simulink model "PenduloRotativoSim"  (R2025a)
settings: Solver=VariableStepAuto  StartTime=0.0  StopTime=4  FixedStep=0.002  RelTol=1e-3  EnableMultiTasking=on
undefined symbols (not defined in the file): K, Ts, x_ic, xp_ic
settings Model: SimulationMode=external  ExtModeTrigDuration=10000  Creator=aluno.engenharia  LastModifiedBy=Mateus
settings SolverCC: AlgebraicLoopSolver=TrustRegion  PositivePriorityOrder=on
settings DebuggingCC: UnconnectedInputMsg=warning  UnconnectedOutputMsg=warning  UnconnectedLineMsg=warning
settings ModelReferenceCC: EnableRefExpFcnMdlSchedulingChecks=on
settings SFSimCC: CustomCodeUndefinedFunction=UseInterfaceOnly
settings RTWCC: SystemTargetFile=quarc_win64.tlc  TemplateMakefile=quarc_default_tmf  GPUComputeCapability=3.5  Description=QUARC Win64 Target
settings STFCustomTargetCC: SystemTargetFile=quarc_win64.tlc  TargetPreCompLibLocation=C:\PROGRA~3\QUARC\lib\2019a\win64\release  TargetLangStandard=C99 (ISO)  MultiwordLength=2048.0  DynamicStringBufferSize=256.0  ConcurrentExecutionCompliant=on  StopOnOverrun=off  DownloadToTarget=on  Debug=off
settings GRTTargetCC: ExtMode=on  ExtModeMexFile=quarc_comm  TargetPreCompLibLocation=C:\PROGRA~3\QUARC\lib\2019a\win64\release  ParMdlRefBuildCompliant=off  CompOptLevelCompliant=off  CombineOutputUpdateFcns=off  MatFileLogging=off  CPPClassGenCompliant=off  GRTInterface=on  UseToolchainInfoCompliant=off

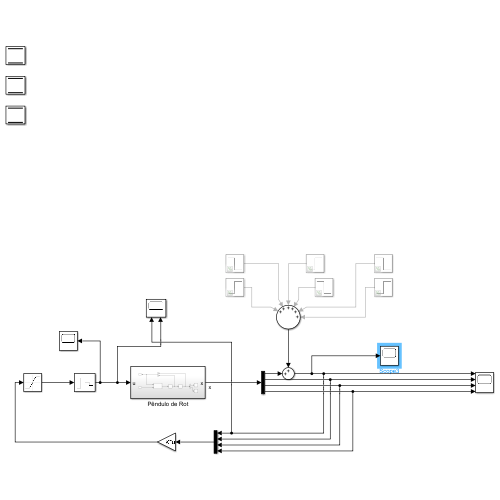
[thumbnail: Simulink's stored preview of the top-level diagram]
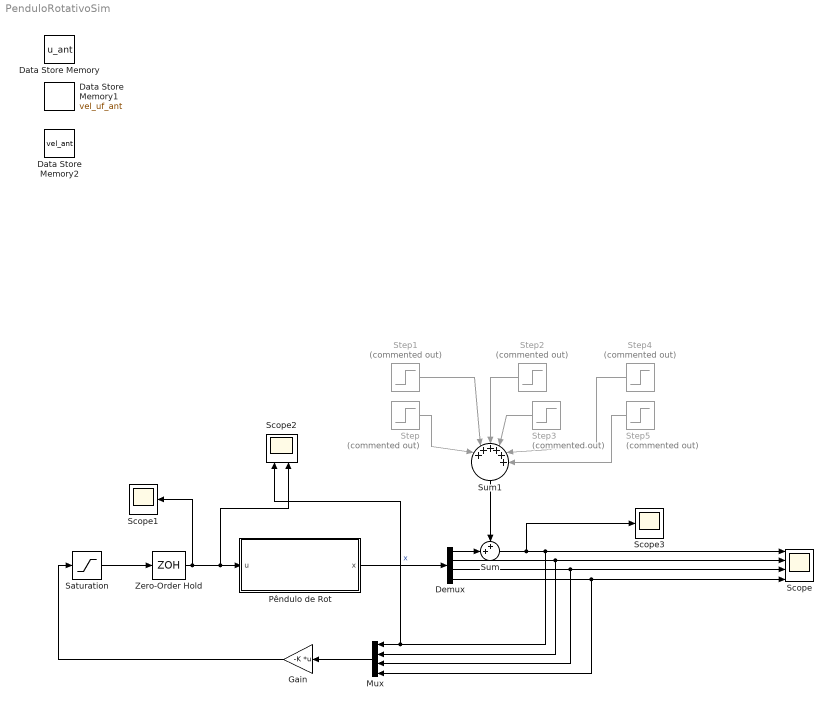
== system PenduloRotativoSim ==
  Data Store Memory : DataStoreMemory  DataStoreName=u_ant  ShowAdditionalParam=off  OutDataTypeStr=double
  Data Store Memory1 : DataStoreMemory  DataStoreName=vel_uf_ant  ReadBeforeWriteMsg=warning  WriteAfterWriteMsg=warning  WriteAfterReadMsg=warning  ShowAdditionalParam=off  OutDataTypeStr=double
  Data Store Memory2 : DataStoreMemory  DataStoreName=vel_ant  ReadBeforeWriteMsg=warning  WriteAfterWriteMsg=warning  WriteAfterReadMsg=warning  ShowAdditionalParam=off  OutDataTypeStr=double
  Demux : Demux
  Gain : Gain  Gain=-K  Multiplication=Matrix(K*u)
  Mux : Mux
  Pêndulo de Rot : Subsystem
  Saturation : Saturate  UpperLimit=12  LowerLimit=-12
  Scope : Scope  NumInputPorts=4
      settings: ActiveDisplayYMinimum=-0.29202531249135588  ActiveDisplayYMaximum=6.0864290081646626
  Scope1 : Scope
      settings: ActiveDisplayYMinimum=-16.513027536482717  ActiveDisplayYMaximum=13.127727482089361  DataLoggingVariableName=ScopeData3
  Scope2 : Scope  NumInputPorts=2
      settings: ActiveDisplayYMinimum=-13.721058256878093  ActiveDisplayYMaximum=11.6029022738507  DataLoggingVariableName=ScopeData4
  Scope3 : Scope
      settings: ActiveDisplayYMinimum=-0.29202531249135588  ActiveDisplayYMaximum=6.0864290081646626  DataLoggingVariableName=ScopeData5
  Step : Step  Commented=on  After=pi/10  SampleTime=0
  Step1 : Step  Commented=on  Time=1.2  After=-pi/10  SampleTime=0
  Step2 : Step  Commented=on  Time=2.5  After=pi/5  SampleTime=0
  Step3 : Step  Commented=on  Time=2.7  After=-pi/5  SampleTime=0
  Step4 : Step  Commented=on  Time=4  After=-pi/5  SampleTime=0
  Step5 : Step  Commented=on  Time=4.2  After=pi/5  SampleTime=0
  Sum : Sum  Inputs=++|
  Sum1 : Sum  Inputs=|++++++
  Zero-Order Hold : ZeroOrderHold  SampleTime=Ts
  wires:
  Gain/1 -> Saturation/1
  Demux/2 -> Mux/2, Scope/2
  Demux/3 -> Scope/3, Mux/3
  Demux/4 -> Scope/4, Mux/4
  Saturation/1 -> Zero-Order Hold/1
  Pêndulo de Rot/1(x) -> Demux/1  "x"
  Demux/1 -> Sum/2
  Step/1 -> Sum1/1
  Sum/1 -> Scope3/1, Scope2/1, Mux/1, Scope/1
  Mux/1 -> Gain/1
  Sum1/1 -> Sum/1
  Step1/1 -> Sum1/2
  Zero-Order Hold/1 -> Scope2/2, Pêndulo de Rot/1(u), Scope1/1
  Step3/1 -> Sum1/4
  Step2/1 -> Sum1/3
  Step4/1 -> Sum1/5
  Step5/1 -> Sum1/6

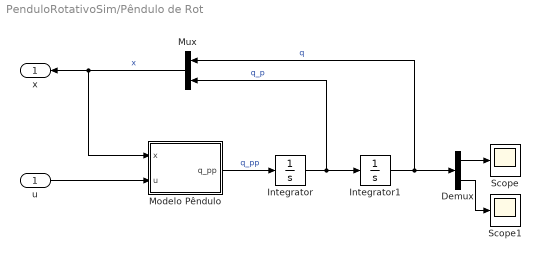
== system PenduloRotativoSim/Pêndulo de Rot ==
  u : Inport
  Demux : Demux  Outputs=2
  Integrator : Integrator  InitialCondition=xp_ic
  Integrator1 : Integrator  InitialCondition=x_ic
  Modelo Pêndulo : MATLAB Function  TreatAsAtomicUnit=on
  Mux : Mux  Inputs=2
  Scope : Scope
      settings: ActiveDisplayYMinimum=-4.469489019623639  ActiveDisplayYMaximum=6.9006379196709613
  Scope1 : Scope
      settings: ActiveDisplayYMinimum=-4.469489019623639  ActiveDisplayYMaximum=6.9006379196709613  DataLoggingVariableName=ScopeData2
  x : Outport
  wires:
  Mux/1 -> x/1, Modelo Pêndulo/1(x)  "x"
  Modelo Pêndulo/1(q_pp) -> Integrator/1  "q_pp"
  u/1 -> Modelo Pêndulo/2(u)
  Integrator/1 -> Mux/2, Integrator1/1  "q_p"
  Integrator1/1 -> Mux/1, Demux/1  "q"
  Demux/1 -> Scope/1
  Demux/2 -> Scope1/1

== matlab function PenduloRotativoSim/Pêndulo de Rot/Modelo Pêndulo ==
  data: x input; q_pp output; u input
function q_pp = fcn(x,u)

th0_  = x(1);
th1_ = x(2);
th0_p  = x(3);
th1_p = x(4);


% Matrizes modelo forma geral (reduziada)
M = function_M_Rot();
V = function_V_Rot(th0_p, th1_p);
G = function_G_Rot(th0_);
P = function_P_Rot();

q_pp = M^-1*(P*u-V-G);
